simulink model "dual_quaternion_library"  (R2017b)
settings: Solver=VariableStepAuto  StartTime=0.0  StopTime=10.0  RelTol=1e-3  EnableMultiTasking=on
settings Model: Creator=viav_gi  LastModifiedBy=hazr_sh
settings OptimizationCC: LifeSpan=inf
settings DebuggingCC: SFUnexpectedBacktrackingDiag=warning  SFNoUnconditionalDefaultTransitionDiag=warning  SFExecutionAtInitializationDiag=none
settings CodeAppCC: StateflowObjectComments=on
settings GRTTargetCC: TargetLangStandard=C89/C90 (ANSI)  GeneratePreprocessorConditionals=Disable all
settings ConfigComp: CovMetricSettings=dw  CovHtmlReporting=on  CovSaveCumulativeToWorkspaceVar=on  CovSaveSingleToWorkspaceVar=on  CovExternalEMLEnable=off

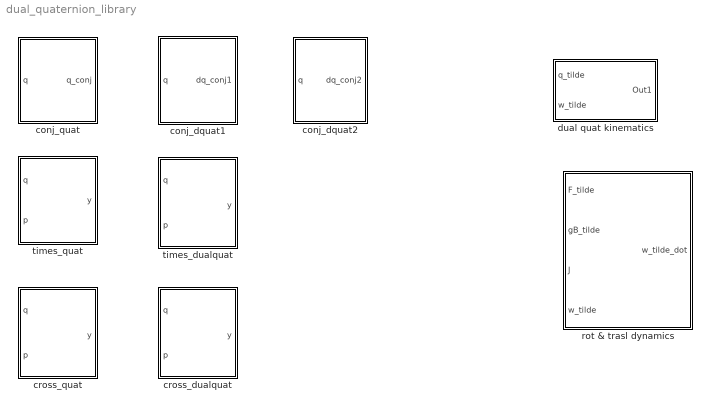
== system dual_quaternion_library ==
  conj_dquat1 : MATLAB Function  TreatAsAtomicUnit=on
  conj_dquat2 : MATLAB Function  TreatAsAtomicUnit=on
  conj_quat : MATLAB Function  TreatAsAtomicUnit=on
  cross_dualquat : MATLAB Function  TreatAsAtomicUnit=on
  cross_quat : MATLAB Function  TreatAsAtomicUnit=on
  dual quat kinematics : Subsystem
  rot & trasl dynamics : Subsystem
  times_dualquat : MATLAB Function  TreatAsAtomicUnit=on
  times_quat : MATLAB Function  TreatAsAtomicUnit=on

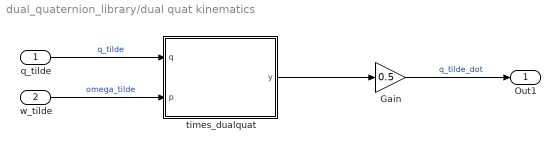
== system dual_quaternion_library/dual quat kinematics ==
  q_tilde : Inport
  w_tilde : Inport  Port=2
  Gain : Gain  Gain=0.5
  times_dualquat : MATLAB Function  TreatAsAtomicUnit=on
  Out1 : Outport
  wires:
  q_tilde/1 -> times_dualquat/1(q)  "q_tilde"
  w_tilde/1 -> times_dualquat/2(p)  "omega_tilde"
  times_dualquat/1(y) -> Gain/1
  Gain/1 -> Out1/1  "q_tilde_dot"

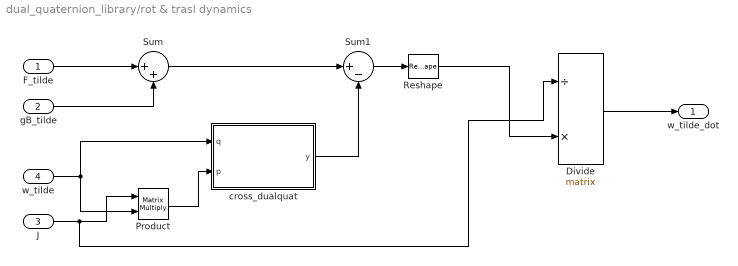
== system dual_quaternion_library/rot & trasl dynamics ==
  F_tilde : Inport
  gB_tilde : Inport  Port=2
  J : Inport  Port=3
  w_tilde : Inport  Port=4
  Divide : Product  Inputs=/*  Multiplication=Matrix(*)
  Product : Product  Multiplication=Matrix(*)
  Reshape : Reshape  OutputDimensionality=Column vector (2-D)
  Sum : Sum  Inputs=|++
  Sum1 : Sum  Inputs=|+-
  cross_dualquat : MATLAB Function  TreatAsAtomicUnit=on
  w_tilde_dot : Outport
  wires:
  F_tilde/1 -> Sum/1
  gB_tilde/1 -> Sum/2
  J/1 -> Divide/1, Product/1
  w_tilde/1 -> cross_dualquat/1(q), Product/2
  Sum/1 -> Sum1/1
  cross_dualquat/1(y) -> Sum1/2
  Divide/1 -> w_tilde_dot/1
  Sum1/1 -> Reshape/1
  Reshape/1 -> Divide/2
  Product/1 -> cross_dualquat/2(p)

== matlab function dual_quaternion_library/cross_dualquat ==
  data: q input; y output; p input
function y = cross_dualquat(q,p)
% Dual Quaternion Cross Product

q1= q(1:4);
q10= q1(4);
q1vect= q1(1:3);

p1= p(1:4);
p10= p1(4);
p1vect= p1(1:3);

q2= q(5:8);
q20= q2(4);
q2vect= q2(1:3);

p2= p(5:8);
p20= p2(4);
p2vect= p2(1:3);

y1= [q10.*p1vect + p10.*q1vect + cross(q1vect, p1vect); 0];
y2= [q10.*p2vect + p20.*q1vect + cross(q1vect, p2vect); 0];
y3= [q20.*p1vect + p10.*q2vect + cross(q2vect, p1vect); 0];

y= [y1; y2+y3];

== matlab function dual_quaternion_library/conj_quat ==
  data: q input; q_conj output
function q_conj = conj_quat(q)
%Unit quaternion conjugation

q0= q(4);
q_vect= q(1:3);

q_conj = [-q_vect; q0];
end

== matlab function dual_quaternion_library/times_quat ==
  data: q input; y output; p input
function y = times_quat(q,p)
% Quaternion multiplication 

q0= q(4);
p0= p(4);

q_vect= q(1:3);
p_vect= p(1:3);


y = [q0.*p_vect + p0.*q_vect + cross(q_vect, p_vect); ...
    q0*p0 - dot(q_vect,p_vect)];

== matlab function dual_quaternion_library/times_dualquat ==
  data: q input; y output; p input
function y = times_dualquat(q,p)
% Dual Quaternion Cross Product

q1= q(1:4);
q10= q1(4);
q1vect= q1(1:3);

p1= p(1:4);
p10= p1(4);
p1vect= p1(1:3);

q2= q(5:8);
q20= q2(4);
q2vect= q2(1:3);

p2= p(5:8);
p20= p2(4);
p2vect= p2(1:3);

y1= [q10.*p1vect + p10.*q1vect + cross(q1vect, p1vect); ...
    q10*p10 - sum(q1vect.*p1vect,1)];
y2= [q10.*p2vect + p20.*q1vect + cross(q1vect, p2vect); ...
    q10*p20 - sum(q1vect.*p2vect,1)];
y3= [q20.*p1vect + p10.*q2vect + cross(q2vect, p1vect); ...
    q20*p10 - sum(q2vect.*p1vect,1)];

y= [y1; y2+y3];

== matlab function dual_quaternion_library/dual quat kinematics/times_dualquat ==
  data: q input; y output; p input
function y = times_dualquat(q,p)
% Dual Quaternion Cross Product

q1= q(1:4);
q10= q1(4);
q1vect= q1(1:3);

p1= p(1:4);
p10= p1(4);
p1vect= p1(1:3);

q2= q(5:8);
q20= q2(4);
q2vect= q2(1:3);

p2= p(5:8);
p20= p2(4);
p2vect= p2(1:3);

y1= [q10.*p1vect + p10.*q1vect + cross(q1vect, p1vect); ...
    q10*p10 - sum(q1vect.*p1vect,1)];
y2= [q10.*p2vect + p20.*q1vect + cross(q1vect, p2vect); ...
    q10*p20 - sum(q1vect.*p2vect,1)];
y3= [q20.*p1vect + p10.*q2vect + cross(q2vect, p1vect); ...
    q20*p10 - sum(q2vect.*p1vect,1)];

y= [y1; y2+y3];

== matlab function dual_quaternion_library/cross_quat ==
  data: q input; y output; p input
function y = cross_quat(q, p)
% Quaternion Cross Product

q4= q(4);
p4= p(4);

q_vect= q(1:3);
p_vect= p(1:3);

y = [q4.*p_vect + p4.*q_vect - cross(q_vect, p_vect); q4*p4 - dot(q_vect,p_vect)];
end

== matlab function dual_quaternion_library/conj_dquat1 ==
  data: q input; dq_conj1 output
function dq_conj1 = conj_dquat1(q)
%Dual quaternion conjugation (q_r^* + q_d^*e)

q1= q(1:4);
q10= q1(4);
q1vect= q1(1:3);

q2= q(5:8);
q20= q2(4);
q2vect= q2(1:3);

dq_conj1 = [-q1_vect; q10; -q2_vect; q20];

== matlab function dual_quaternion_library/conj_dquat2 ==
  data: q input; dq_conj2 output
function dq_conj2 = conj_dquat2(q)
%Dual quaternion conjugation (q_r^* - q_d^*e)

q1= q(1:4);
q10= q1(4);
q1vect= q1(1:3);

q2= q(5:8);
q20= q2(4);
q2vect= q2(1:3);

dq_conj2 = [-q1_vect; q10; q2_vect; -q20];

== matlab function dual_quaternion_library/rot & trasl dynamics/cross_dualquat ==
  data: q input; y output; p input
function y = cross_dualquat(q,p)
% Dual Quaternion Cross Product

q1= q(1:4);
q10= q1(4);
q1vect= q1(1:3);

p1= p(1:4);
p10= p1(4);
p1vect= p1(1:3);

q2= q(5:8);
q20= q2(4);
q2vect= q2(1:3);

p2= p(5:8);
p20= p2(4);
p2vect= p2(1:3);

y1= [q10.*p1vect + p10.*q1vect + cross(q1vect, p1vect); 0];
y2= [q10.*p2vect + p20.*q1vect + cross(q1vect, p2vect); 0];
y3= [q20.*p1vect + p10.*q2vect + cross(q2vect, p1vect); 0];

y= [y1; y2+y3];
